simulink library "motor_characteristic"  (R2020b)
settings: Solver=VariableStepAuto  StartTime=0.0  StopTime=10.0  RelTol=1e-3
values from neighbouring files (symbols this model uses):
  motor_power = motor_data(2:12,2:end)    [init.m]
  motor_speed = motor_data(2:12,1)    [init.m]
  motor_torque = motor_data(1,2:end)    [init.m]
  P_consumer = 1050    [init.m]
settings Model: Creator=janbantle  LastModifiedBy=vanes

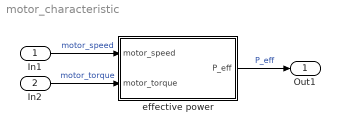
== system motor_characteristic ==
  In1 : Inport
  In2 : Inport  Port=2
  effective power : Subsystem
  Out1 : Outport
  wires:
  In1/1 -> effective power/1(motor_speed)  "motor_speed"
  In2/1 -> effective power/2(motor_torque)  "motor_torque"
  effective power/1(P_eff) -> Out1/1  "P_eff"

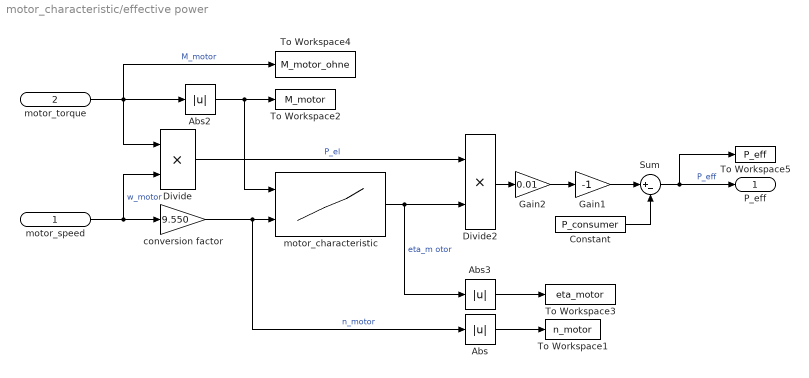
== system motor_characteristic/effective power ==
  motor_speed : Inport
  motor_torque : Inport  Port=2
  Abs : Abs
  Abs2 : Abs
  Abs3 : Abs
  Constant : Constant  Value=P_consumer
  Divide : Product  Inputs=**
  Divide2 : Product  Inputs=**
  Gain1 : Gain  Gain=-1
  Gain2 : Gain  Gain=0.01
  Sum : Sum  Inputs=|+-
  To Workspace1 : ToWorkspace  VariableName=n_motor  SampleTime=-1
  To Workspace2 : ToWorkspace  VariableName=M_motor  SampleTime=-1
  To Workspace3 : ToWorkspace  VariableName=eta_motor  SampleTime=-1
  To Workspace4 : ToWorkspace  VariableName=M_motor_ohne  SampleTime=-1
  To Workspace5 : ToWorkspace  VariableName=P_eff  SampleTime=-1
  conversion factor : Gain  Gain=9.550
  motor_characteristic : Lookup_n-D  BreakpointsForDimension1=motor_speed  BreakpointsForDimension2=motor_torque  BreakpointsForDimension3=[5, 7]  IndexSearchMethod=Linear search  Table=motor_power  InternalRulePriority=Speed  RndMeth=Simplest  InputSameDT=on
      settings: InputPortMap=u0,u1
  P_eff : Outport
  wires:
  Gain1/1 -> Sum/1
  Abs2/1 -> motor_characteristic/1, To Workspace2/1
  Abs/1 -> To Workspace1/1
  Sum/1 -> P_eff/1, To Workspace5/1  "P_eff"
  Constant/1 -> Sum/2
  Divide/1 -> Divide2/1  "P_el"
  motor_characteristic/1 -> Divide2/2, Abs3/1  "eta_m otor"
  motor_speed/1 -> conversion factor/1, Divide/2  "w_motor"
  motor_torque/1 -> To Workspace4/1, Divide/1, Abs2/1  "M_motor"
  conversion factor/1 -> motor_characteristic/2, Abs/1  "n_motor"
  Divide2/1 -> Gain2/1
  Gain2/1 -> Gain1/1
  Abs3/1 -> To Workspace3/1
